simulink model "SHIP_DOWN_matlab_2017"  (R2018b)
settings: Solver=ode8  StartTime=0.0  StopTime=1.5  RelTol=1e-3
undefined symbols (not defined in the file): Cout_c, Cout_r, Cvh_c, Cvh_r, DiscIntNeverNeededParam, f, L1_l, L1_r, Lvh_l, Lvh_r, R_out, Uout, Uvh
libraries: powerlib x13, powerlib_meascontrol x8, simulink x2, simulink_extras x1
settings Model: Creator=Anton  LastModifiedBy=VID Company
settings SFSimCC: SimUseLocalCustomCode=off
settings RTWCC: RTWUseLocalCustomCode=off
settings CodeAppCC: StateflowObjectComments=on
settings SimscapeCC: SimscapeNormalizeSystem=off

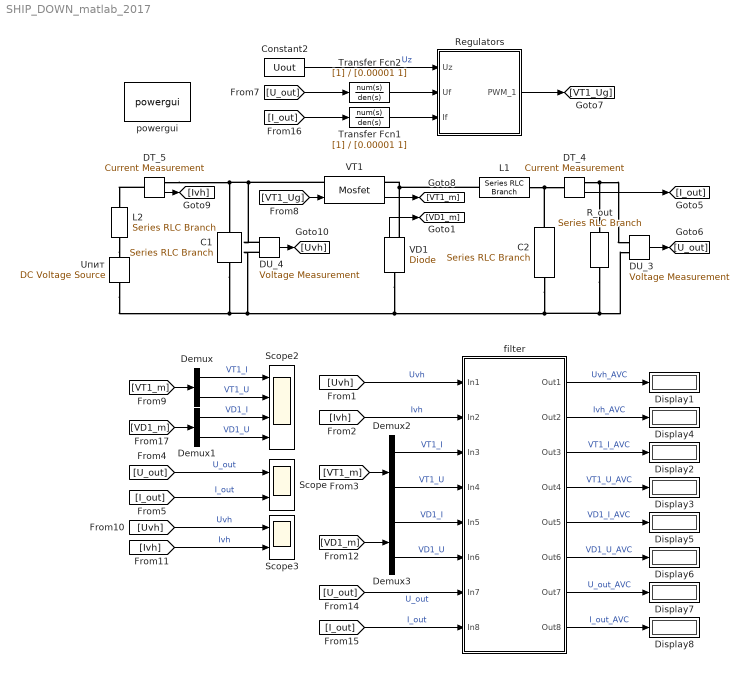
== system SHIP_DOWN_matlab_2017 ==
  C1 : powerlib/Elements/Series RLC Branch  LConnTagsString=__new0  RConnTagsString=__new0  BranchType=RC  Resistance=Cvh_r  Inductance=1e-3  SetiL0=off  InitialCurrent=0  Capacitance=Cvh_c  Setx0=on  InitialVoltage=Uvh  Measurements=Branch voltage
      settings: SourceProductName=Simscape Electrical
  C2 : powerlib/Elements/Series RLC Branch  LConnTagsString=__new0  RConnTagsString=__new0  BranchType=RC  Resistance=Cout_r  Inductance=1e-3  SetiL0=off  InitialCurrent=0  Capacitance=Cout_c  Setx0=on  InitialVoltage=0  Measurements=Branch voltage
      settings: SourceProductName=Simscape Electrical
  Constant2 : Constant  Value=Uout
  DT_4 : powerlib/Measurements/Current Measurement  PhasorSimulation=off  OutputType=Complex  PSBequivalent=0
      settings: SourceProductName=Simscape Electrical
  DT_5 : powerlib/Measurements/Current Measurement  PhasorSimulation=off  OutputType=Complex  PSBequivalent=0
      settings: SourceProductName=Simscape Electrical
  DU_3 : powerlib/Measurements/Voltage Measurement  PhasorSimulation=off  OutputType=Complex  PSBequivalent=0
      settings: SourceProductName=Simscape Electrical
  DU_4 : powerlib/Measurements/Voltage Measurement  PhasorSimulation=off  OutputType=Complex  PSBequivalent=0
      settings: SourceProductName=Simscape Electrical
  Demux{,1..3} (4 alike) : Demux  Outputs=2
  Display{1..8} (8 alike) : Display
  L1 : powerlib/Elements/Series RLC Branch  LConnTagsString=__new0  RConnTagsString=__new0  BranchType=RL  Resistance=L1_r  Inductance=L1_l  SetiL0=off  InitialCurrent=0  Capacitance=1e-6  Setx0=off  InitialVoltage=0  Measurements=None
      settings: SourceProductName=Simscape Electrical
  L2 : powerlib/Elements/Series RLC Branch  LConnTagsString=__new0  RConnTagsString=__new0  BranchType=RL  Resistance=Lvh_r  Inductance=Lvh_l  SetiL0=off  InitialCurrent=0  Capacitance=1e-6  Setx0=off  InitialVoltage=0  Measurements=None
      settings: SourceProductName=Simscape Electrical
  R_out : powerlib/Elements/Series RLC Branch  LConnTagsString=__new0  RConnTagsString=__new0  BranchType=R  Resistance=R_out  Inductance=1e-3  SetiL0=off  InitialCurrent=0  Capacitance=1e-6  Setx0=off  InitialVoltage=0  Measurements=None
      settings: SourceProductName=Simscape Electrical
  Regulators : Subsystem
  Scope : Scope  NumInputPorts=2
  Scope2 : Scope  NumInputPorts=4
  Scope3 : Scope  NumInputPorts=2
  Transfer Fcn1 : TransferFcn  Denominator=[0.00001 1]
  Transfer Fcn2 : TransferFcn  Denominator=[0.00001 1]
  Uпит : powerlib/Electrical Sources/DC Voltage Source  Amplitude=Uvh  Measurements=None
      settings: SourceProductName=Simscape Electrical
  VD1 : powerlib/Power Electronics/Diode  Ron=0.001  Lon=0  Vf=1  IC=0  UseSnubber=off  Rs=inf  Cs=inf  Measurements=on
      settings: SourceProductName=Simscape Electrical
  VT1 : powerlib/Power Electronics/Mosfet  Ron=10e-3  Lon=inf  Rd=10e-3  Vfd=1  IC=0  Rs=1e5  Cs=inf  Measurements=on
      settings: SourceProductName=Simscape Electrical
  filter : Subsystem
  powergui : powerlib/powergui  Priority=1  SimulationMode=Discrete  SampleTime=1e-6  frequency=60  Iterations=50  frequencyindice=0  Pbase=100e6  ErrMax=1e-4  UnitsV=kV  UnitsW=MW  buscounter=0  FunctionMessages=off  echomessages=off  EnableUseOfTLC=off  CurrentSourceSwitches=off  DisableSnubberDevices=off  DisableRonSwitches=off  DisableVfSwitches=off  DisplayEquations=off  SolverType=Tustin/Backward Euler (TBE)  Interpol=off  ExternalGateDelay=off  methode=off  Ts=100  x0status=blocks  SPID=off  SwTol=0  HookPort=off  RestoreLinks=warning  ResistiveCurrentMeasurement=off  Frange=[0:2:500]  Ylog=off  Xlog=on  ShowGrid=off  save=off  variable=ZData  structure=0  ZoomFFT=off  StartTime=0.0  cycles=1  DisplayStyle=1  fundamental=60  FreqAxis=off  MaxFrequency=1000  frequencyindicesteady=1  RmsSteady=1  display=off
  wires:
  Transfer Fcn2/1 -> Regulators/2(Uf)
  Constant2/1 -> Regulators/1(Uz)  "Uz"
  DT_4/1 -> [I_out]
  DU_3/1 -> [U_out]
  [U_out] -> Scope/1  "U_out"
  [I_out] -> Scope/2  "I_out"
  [U_out] -> Transfer Fcn2/1
  [VT1_Ug] -> VT1/1
  Demux/1 -> Scope2/1  "VT1_I"
  Demux/2 -> Scope2/2  "VT1_U"
  VT1/1 -> [VT1_m]
  [VT1_m] -> Demux/1
  DT_5/1 -> [Ivh]
  DU_4/1 -> [Uvh]
  [Ivh] -> Scope3/2  "Ivh"
  [Uvh] -> Scope3/1  "Uvh"
  filter/3(Out3) -> Display2/1  "VT1_I_AVC"
  Demux2/1 -> filter/3(In3)  "VT1_I"
  Demux2/2 -> filter/4(In4)  "VT1_U"
  filter/4(Out4) -> Display3/1  "VT1_U_AVC"
  [U_out] -> filter/7(In7)  "U_out"
  [I_out] -> filter/8(In8)  "I_out"
  [I_out] -> Transfer Fcn1/1
  VD1/1 -> [VD1_m]
  [VD1_m] -> Demux1/1
  Demux1/1 -> Scope2/3  "VD1_I"
  Demux1/2 -> Scope2/4  "VD1_U"
  [Uvh] -> filter/1(In1)  "Uvh"
  [Ivh] -> filter/2(In2)  "Ivh"
  filter/1(Out1) -> Display1/1  "Uvh_AVC"
  filter/2(Out2) -> Display4/1  "Ivh_AVC"
  [VT1_m] -> Demux2/1
  [VD1_m] -> Demux3/1
  filter/6(Out6) -> Display6/1  "VD1_U_AVC"
  filter/5(Out5) -> Display5/1  "VD1_I_AVC"
  Demux3/1 -> filter/5(In5)  "VD1_I"
  Demux3/2 -> filter/6(In6)  "VD1_U"
  filter/7(Out7) -> Display7/1  "U_out_AVC"
  filter/8(Out8) -> Display8/1  "I_out_AVC"
  Regulators/1(PWM_1) -> [VT1_Ug]
  Transfer Fcn1/1 -> Regulators/3(If)
  connections:
  DT_4/RConn1 -- DU_3/LConn1 -- R_out/LConn1
  C2/LConn1 -- DT_4/LConn1 -- L1/RConn1
  C1/RConn1 -- Uпит/LConn1 -- DU_4/LConn2 -- VD1/LConn1 -- R_out/RConn1 -- DU_3/LConn2 -- C2/RConn1
  L1/LConn1 -- VD1/RConn1 -- VT1/RConn1
  DU_4/LConn1 -- C1/LConn1 -- DT_5/RConn1 -- VT1/LConn1
  L2/LConn1 -- Uпит/RConn1
  DT_5/LConn1 -- L2/RConn1

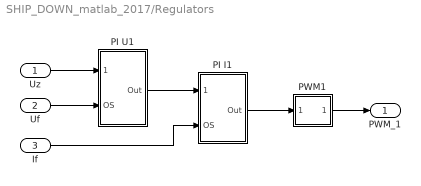
== system SHIP_DOWN_matlab_2017/Regulators ==
  Uz : Inport
  Uf : Inport  Port=2
  If : Inport  Port=3
  PI I1 : Subsystem
  PI U1 : Subsystem
  PWM1 : Subsystem
  PWM_1 : Outport
  wires:
  PWM1/1(CH1) -> PWM_1/1
  PI I1/1(Out) -> PWM1/1(Uz)
  Uz/1 -> PI U1/1(Zad)
  Uf/1 -> PI U1/2(OS)
  PI U1/1(Out) -> PI I1/1(Zad)
  If/1 -> PI I1/2(OS)

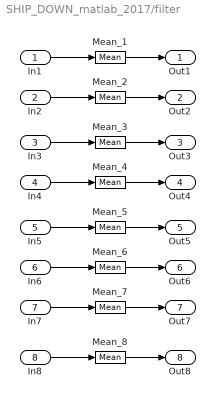
== system SHIP_DOWN_matlab_2017/filter ==
  In1 : Inport
  In2 : Inport  Port=2
  In3 : Inport  Port=3
  In4 : Inport  Port=4
  In5 : Inport  Port=5
  In6 : Inport  Port=6
  In7 : Inport  Port=7
  In8 : Inport  Port=8
  Mean_{1..8} (8 alike) : powerlib_meascontrol/Measurements/Mean  Freq=100  Vinit=0  Ts=0
  Out1 : Outport
  Out2 : Outport  Port=2
  Out3 : Outport  Port=3
  Out4 : Outport  Port=4
  Out5 : Outport  Port=5
  Out6 : Outport  Port=6
  Out7 : Outport  Port=7
  Out8 : Outport  Port=8
  wires:
  In1/1 -> Mean_1/1
  In2/1 -> Mean_2/1
  In3/1 -> Mean_3/1
  In4/1 -> Mean_4/1
  In5/1 -> Mean_5/1
  In6/1 -> Mean_6/1
  In7/1 -> Mean_7/1
  In8/1 -> Mean_8/1
  Mean_1/1 -> Out1/1
  Mean_2/1 -> Out2/1
  Mean_3/1 -> Out3/1
  Mean_4/1 -> Out4/1
  Mean_5/1 -> Out5/1
  Mean_6/1 -> Out6/1
  Mean_8/1 -> Out8/1
  Mean_7/1 -> Out7/1

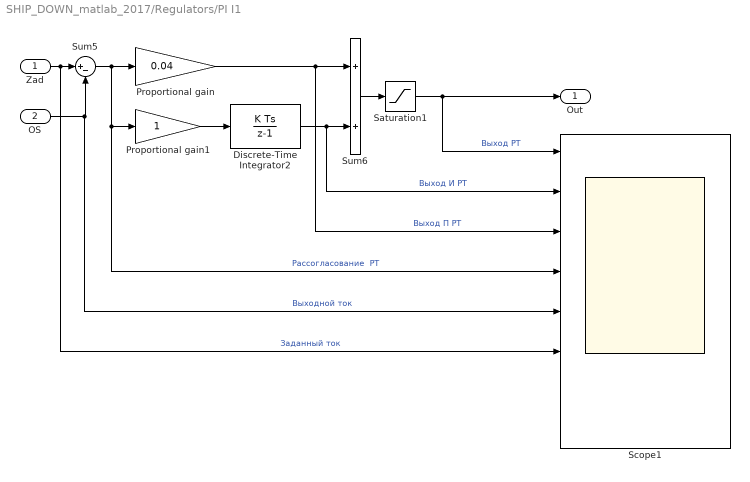
== system SHIP_DOWN_matlab_2017/Regulators/PI I1 ==
  Zad : Inport
  OS : Inport  Port=2
  Discrete-Time Integrator2 : DiscreteIntegrator  SampleTime=-1  LimitOutput=on  UpperSaturationLimit=0.9  LowerSaturationLimit=0  ICPrevOutput=DiscIntNeverNeededParam  ICPrevScaledInput=DiscIntNeverNeededParam
  Proportional gain : Gain  Gain=0.04  SaturateOnIntegerOverflow=on  OutDataTypeStr=Inherit: Same as input  ParamDataTypeStr=Inherit: Same as input
  Proportional gain1 : Gain  SaturateOnIntegerOverflow=on  OutDataTypeStr=Inherit: Same as input  ParamDataTypeStr=Inherit: Same as input
  Saturation1 : Saturate  UpperLimit=0.9  LowerLimit=0
  Scope1 : Scope  NumInputPorts=8
  Sum5 : Sum  Inputs=|+-  SaturateOnIntegerOverflow=on  InputSameDT=on  OutDataTypeStr=Inherit: Same as first input
  Sum6 : Sum  SaturateOnIntegerOverflow=on  InputSameDT=on  OutDataTypeStr=Inherit: Same as first input
  Out : Outport
  wires:
  Proportional gain/1 -> Scope1/3, Sum6/1  "Выход П РТ"
  Discrete-Time Integrator2/1 -> Sum6/2, Scope1/2  "Выход И РТ"
  OS/1 -> Scope1/5, Sum5/2  "Выходной ток"
  Zad/1 -> Scope1/6, Sum5/1  "Заданный ток"
  Sum5/1 -> Proportional gain1/1, Scope1/4, Proportional gain/1  "Рассогласование  РТ"
  Sum6/1 -> Saturation1/1
  Saturation1/1 -> Out/1, Scope1/1  "Выход РТ"
  Proportional gain1/1 -> Discrete-Time Integrator2/1

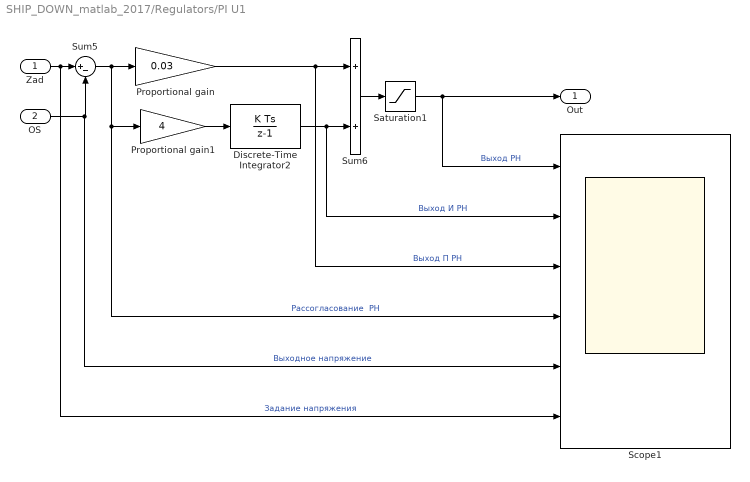
== system SHIP_DOWN_matlab_2017/Regulators/PI U1 ==
  Zad : Inport
  OS : Inport  Port=2
  Discrete-Time Integrator2 : DiscreteIntegrator  SampleTime=-1  LimitOutput=on  UpperSaturationLimit=120  LowerSaturationLimit=0  ICPrevOutput=DiscIntNeverNeededParam  ICPrevScaledInput=DiscIntNeverNeededParam
  Proportional gain : Gain  Gain=0.03  SaturateOnIntegerOverflow=on  OutDataTypeStr=Inherit: Same as input  ParamDataTypeStr=Inherit: Same as input
  Proportional gain1 : Gain  Gain=4  SaturateOnIntegerOverflow=on  OutDataTypeStr=Inherit: Same as input  ParamDataTypeStr=Inherit: Same as input
  Saturation1 : Saturate  UpperLimit=120  LowerLimit=0
  Scope1 : Scope  NumInputPorts=6
  Sum5 : Sum  Inputs=|+-  SaturateOnIntegerOverflow=on  InputSameDT=on  OutDataTypeStr=Inherit: Same as first input
  Sum6 : Sum  SaturateOnIntegerOverflow=on  InputSameDT=on  OutDataTypeStr=Inherit: Same as first input
  Out : Outport
  wires:
  Proportional gain/1 -> Scope1/3, Sum6/1  "Выход П РН"
  Discrete-Time Integrator2/1 -> Sum6/2, Scope1/2  "Выход И РН"
  OS/1 -> Scope1/5, Sum5/2  "Выходное напряжение"
  Zad/1 -> Scope1/6, Sum5/1  "Задание напряжения"
  Sum5/1 -> Proportional gain1/1, Scope1/4, Proportional gain/1  "Рассогласование  РН"
  Sum6/1 -> Saturation1/1
  Saturation1/1 -> Out/1, Scope1/1  "Выход РН"
  Proportional gain1/1 -> Discrete-Time Integrator2/1

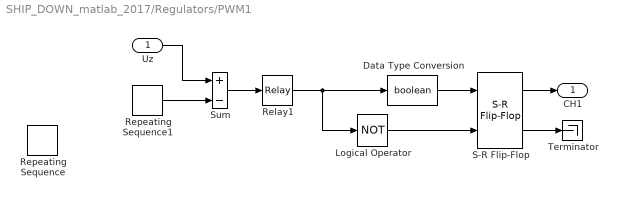
== system SHIP_DOWN_matlab_2017/Regulators/PWM1 ==
  Uz : Inport
  Data Type Conversion : DataTypeConversion  OutDataTypeStr=boolean
  Logical Operator : Logic  Operator=NOT  AllPortsSameDT=off  OutDataTypeStr=boolean
  Relay1 : Relay  OnSwitchValue=0.01  OffSwitchValue=-0.01
  Repeating Sequence : simulink/Sources/Repeating Sequence  rep_seq_t=[0 0.00025]  rep_seq_y=[0 1]
  Repeating Sequence1 : simulink/Sources/Repeating Sequence  rep_seq_t="[0  (1/(2*f)) (1/f)]"  rep_seq_y=[0 1 0]
  S-R Flip-Flop : simulink_extras/Flip Flops/S-R Flip-Flop  initial_condition=0
  Sum : Sum  Inputs=+-
  Terminator : Terminator
  CH1 : Outport
  wires:
  S-R Flip-Flop/1 -> CH1/1
  Data Type Conversion/1 -> S-R Flip-Flop/1
  Logical Operator/1 -> S-R Flip-Flop/2
  Relay1/1 -> Logical Operator/1, Data Type Conversion/1
  Uz/1 -> Sum/1
  Sum/1 -> Relay1/1
  S-R Flip-Flop/2 -> Terminator/1
  Repeating Sequence1/1 -> Sum/2
